simulink model "actividad1simulink"  (R2021a)
settings: Solver=ode1  StartTime=0.0  StopTime=100  FixedStep=0.001  RelTol=1e-3
settings Model: Creator=Agus  LastModifiedBy=Agus

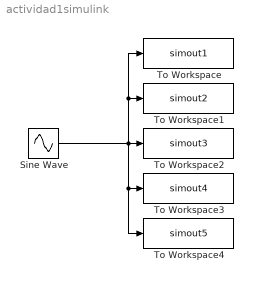
== system actividad1simulink ==
  Sine Wave : Sin  Frequency=2*pi  SampleTime=0
  To Workspace : ToWorkspace  VariableName=simout1  SaveFormat=Timeseries  SampleTime=-1
  To Workspace1 : ToWorkspace  VariableName=simout2  SaveFormat=Timeseries  SampleTime=0.51
  To Workspace2 : ToWorkspace  VariableName=simout3  SaveFormat=Timeseries  SampleTime=0.5
  To Workspace3 : ToWorkspace  VariableName=simout4  SaveFormat=Timeseries  SampleTime=0.49
  To Workspace4 : ToWorkspace  VariableName=simout5  SaveFormat=Timeseries  SampleTime=0.1
  wires:
  Sine Wave/1 -> To Workspace4/1, To Workspace3/1, To Workspace/1, To Workspace1/1, To Workspace2/1
